simulink model "stack_parameters_estimation_standalone"  (R2023a)
settings: Solver=VariableStepAuto  StartTime=0.0  StopTime=10.0  RelTol=1e-3
settings Model: Creator=adrian.taveras  LastModifiedBy=adrian.taveras

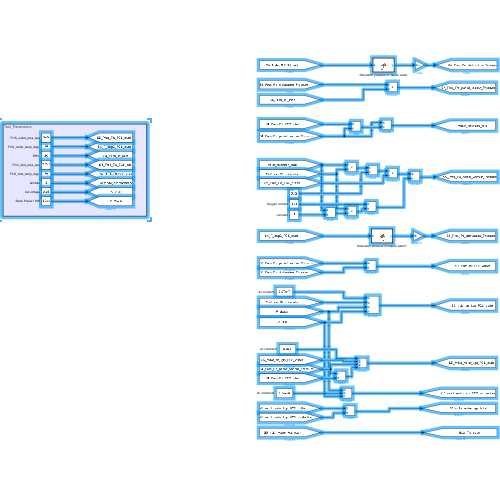
[thumbnail: Simulink's stored preview of the top-level diagram]
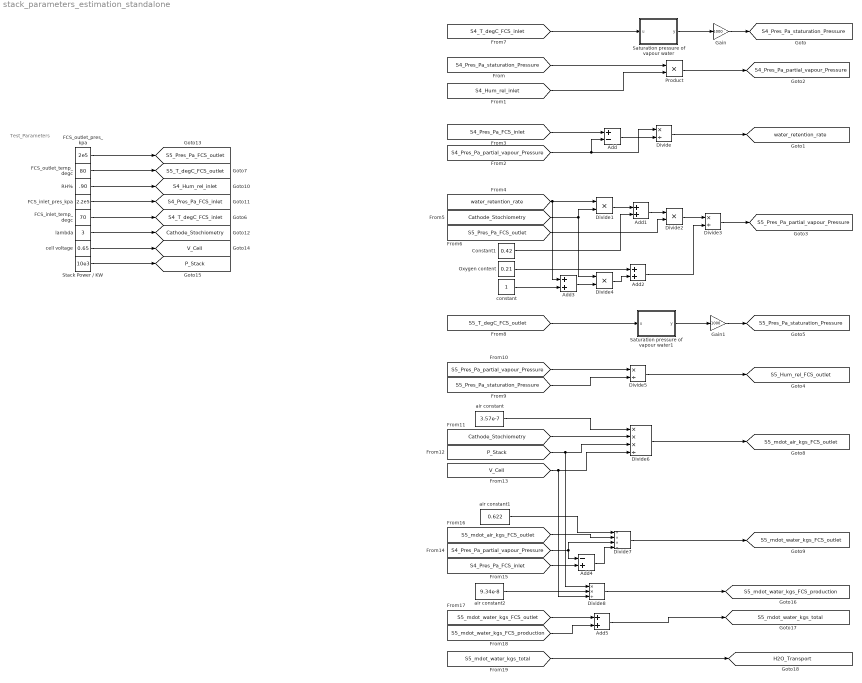
== system stack_parameters_estimation_standalone ==
  note: Test_Parameters
  Add : Sum  Inputs=+-
  Add{1..3,5} (4 alike) : Sum
  Add4 : Sum  Inputs=-+
  Constant1 : Constant  Value=0.42
  Divide : Product  Inputs=*/
  Divide1 : Product  Inputs=**
  Divide2 : Product  Inputs=**
  Divide3 : Product  Inputs=*/
  Divide4 : Product  Inputs=**
  Divide5 : Product  Inputs=*/
  Divide6 : Product  Inputs=***/
  Divide7 : Product  Inputs=***/
  Divide8 : Product  Inputs=**/
  FCS_inlet_pres_kpa : Constant  Value=2.2e5
  FCS_inlet_temp_degc : Constant  Value=70
  FCS_outlet_pres_kpa : Constant  Value=2e5
  FCS_outlet_temp_degc : Constant  Value=80
  Gain : Gain  Gain=1000
  Gain1 : Gain  Gain=1000
  Oxygen content : Constant  Value=0.21
  Product : Product
  RH% : Constant  Value=.90
  Saturation pressure of vapour water : MATLAB Function  TreatAsAtomicUnit=on
  Saturation pressure of vapour water1 : MATLAB Function  TreatAsAtomicUnit=on
  Stack Power / KW : Constant  Value=10e3
  air constant : Constant  Value=3.57e-7
  air constant1 : Constant  Value=0.622
  air constant2 : Constant  Value=9.34e-8
  cell voltage : Constant  Value=0.65
  constant : Constant
  lambda : Constant  Value=3
  tag scope: Cathode_Stochiometry=global, H2O_Transport=global, P_Stack=global, S4_Hum_rel_inlet=global, S4_Pres_Pa_FCS_inlet=global, S4_Pres_Pa_partial_vapour_Pressure=global, S4_Pres_Pa_staturation_Pressure=global, S4_T_degC_FCS_inlet=global, S5_Hum_rel_FCS_outlet=global, S5_Pres_Pa_FCS_outlet=global, S5_Pres_Pa_partial_vapour_Pressure=global, S5_Pres_Pa_staturation_Pressure=global, S5_T_degC_FCS_outlet=global, S5_mdot_air_kgs_FCS_outlet=global, S5_mdot_water_kgs_FCS_outlet=global, S5_mdot_water_kgs_FCS_production=global, S5_mdot_water_kgs_total=global, V_Cell=global, water_retention_rate=global
  wires:
  Saturation pressure of vapour water/1(y) -> Gain/1
  [S4_T_degC_FCS_inlet] -> Saturation pressure of vapour water/1(u)
  Gain/1 -> [S4_Pres_Pa_staturation_Pressure]
  [S4_Pres_Pa_staturation_Pressure] -> Product/1
  [S4_Hum_rel_inlet] -> Product/2
  Product/1 -> [S4_Pres_Pa_partial_vapour_Pressure]
  [S4_Pres_Pa_FCS_inlet] -> Add/1
  [S4_Pres_Pa_partial_vapour_Pressure] -> Divide/1, Add/2
  Add/1 -> Divide/2
  Divide/1 -> [water_retention_rate]
  [Cathode_Stochiometry] -> Divide4/1, Divide1/2
  [water_retention_rate] -> Divide1/1, Add3/1
  Divide1/1 -> Add1/1
  Constant1/1 -> Add1/2
  Add1/1 -> Divide2/1
  [S5_Pres_Pa_FCS_outlet] -> Divide2/2
  Divide2/1 -> Divide3/1
  Oxygen content/1 -> Add2/1
  constant/1 -> Add3/2
  Add3/1 -> Divide4/2
  Divide4/1 -> Add2/2
  Add2/1 -> Divide3/2
  Gain1/1 -> [S5_Pres_Pa_staturation_Pressure]
  [S5_T_degC_FCS_outlet] -> Saturation pressure of vapour water1/1(u)
  Saturation pressure of vapour water1/1(y) -> Gain1/1
  FCS_inlet_temp_degc/1 -> [S4_T_degC_FCS_inlet]
  [S5_Pres_Pa_partial_vapour_Pressure] -> Divide5/1
  [S5_Pres_Pa_staturation_Pressure] -> Divide5/2
  Divide5/1 -> [S5_Hum_rel_FCS_outlet]
  FCS_outlet_temp_degc/1 -> [S5_T_degC_FCS_outlet]
  [V_Cell] -> Divide8/3, Divide6/4
  [P_Stack] -> Divide8/1, Divide6/3
  air constant/1 -> Divide6/1
  [Cathode_Stochiometry] -> Divide6/2
  Divide6/1 -> [S5_mdot_air_kgs_FCS_outlet]
  RH%/1 -> [S4_Hum_rel_inlet]
  FCS_inlet_pres_kpa/1 -> [S4_Pres_Pa_FCS_inlet]
  lambda/1 -> [Cathode_Stochiometry]
  FCS_outlet_pres_kpa/1 -> [S5_Pres_Pa_FCS_outlet]
  cell voltage/1 -> [V_Cell]
  Stack Power / KW/1 -> [P_Stack]
  air constant1/1 -> Divide7/1
  [S4_Pres_Pa_partial_vapour_Pressure] -> Divide7/3, Add4/1
  [S4_Pres_Pa_FCS_inlet] -> Add4/2
  Add4/1 -> Divide7/4
  Divide7/1 -> [S5_mdot_water_kgs_FCS_outlet]
  air constant2/1 -> Divide8/2
  Divide8/1 -> [S5_mdot_water_kgs_FCS_production]
  Divide3/1 -> [S5_Pres_Pa_partial_vapour_Pressure]
  [S5_mdot_air_kgs_FCS_outlet] -> Divide7/2
  [S5_mdot_water_kgs_FCS_outlet] -> Add5/1
  [S5_mdot_water_kgs_FCS_production] -> Add5/2
  Add5/1 -> [S5_mdot_water_kgs_total]
  [S5_mdot_water_kgs_total] -> [H2O_Transport]

== matlab function stack_parameters_estimation_standalone/Saturation pressure of vapour water ==
  data: u input; y output
function y = fcn(u)

y =  0.61121 * exp((18.678 - (u / 234.5)) * (u / (257.14 + u)));;

== matlab function stack_parameters_estimation_standalone/Saturation pressure of vapour water1 ==
  data: u input; y output
function y = fcn(u)

y =  0.61121 * exp((18.678 - (u / 234.5)) * (u / (257.14 + u)));;
